simulink model "CommandBRobustesse"  (R2018b)
settings: Solver=VariableStepAuto  StartTime=0.0  StopTime=10.0  RelTol=1e-3
libraries: cstblocks x4
settings Model: Creator=olavoie  LastModifiedBy=olavoie

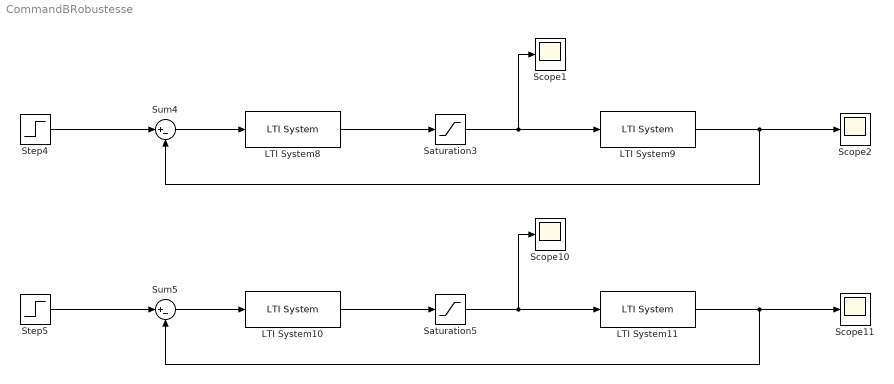
== system CommandBRobustesse ==
  LTI System10 : cstblocks/LTI System  sys=Cx  IC=[]
  LTI System11 : cstblocks/LTI System  sys=Px2  IC=[]
  LTI System8 : cstblocks/LTI System  sys=Cx  IC=[]
  LTI System9 : cstblocks/LTI System  sys=Px1  IC=[]
  Saturation3 : Saturate  UpperLimit=110  LowerLimit=-110
  Saturation5 : Saturate  UpperLimit=110  LowerLimit=-110
  Scope{1..2,10..11} (4 alike) : Scope
  Step4 : Step  Time=0  After=0.5  SampleTime=0  VectorParams1D=off
  Step5 : Step  Time=0  After=0.5  SampleTime=0  VectorParams1D=off
  Sum4 : Sum  Inputs=|+-
  Sum5 : Sum  Inputs=|+-
  wires:
  LTI System11/1 -> Sum5/2, Scope11/1
  Saturation5/1 -> Scope10/1, LTI System11/1
  LTI System10/1 -> Saturation5/1
  Step5/1 -> Sum5/1
  LTI System9/1 -> Scope2/1, Sum4/2
  Sum4/1 -> LTI System8/1
  Saturation3/1 -> Scope1/1, LTI System9/1
  Sum5/1 -> LTI System10/1
  Step4/1 -> Sum4/1
  LTI System8/1 -> Saturation3/1
